simulink model "hamburger"  (R2021a)
settings: Solver=FixedStepAuto  StartTime=0.0  StopTime=150  FixedStep=0.1  RelTol=1e-3
settings Model: Creator=templ  LastModifiedBy=templ
settings DataIOCC: ReturnWorkspaceOutputs=off

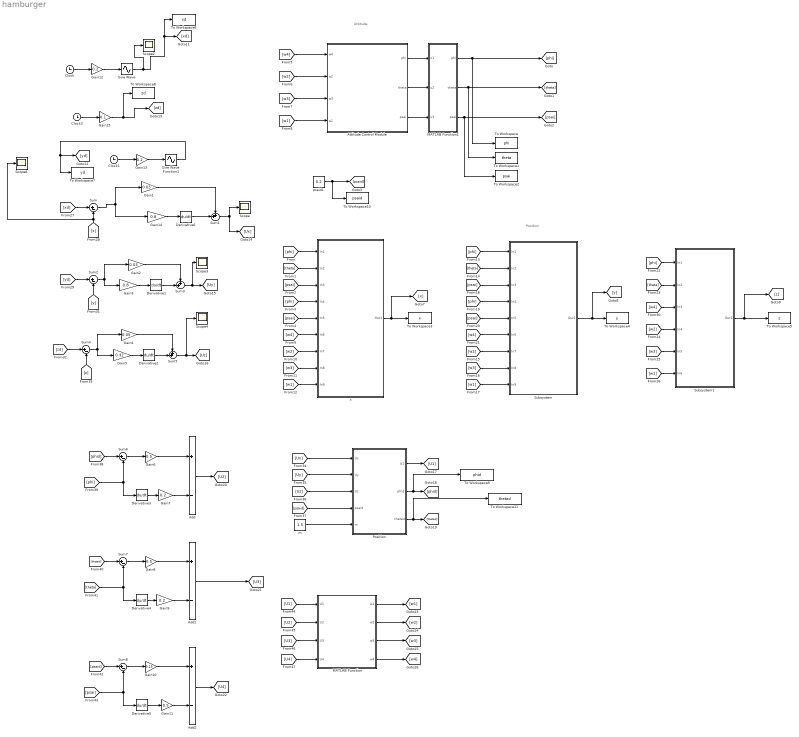
== system hamburger ==
  note: Attitude
  note: Position
  Add : Sum  Inputs=+-
  Add1 : Sum  Inputs=+-
  Add2 : Sum  Inputs=+-
  Attitude Control Module : Subsystem
  Clock : Clock
  Clock1 : Clock
  Clock3 : Clock
  Derivative{1..6} (6 alike) : Derivative
  Gain1 : Gain  Gain=0.03
  Gain10 : Gain  Gain=0.25
  Gain11 : Gain  Gain=0.5
  Gain{7,9,12..13} (4 alike) : Gain  Gain=0.2
  Gain14 : Gain  Gain=0.8
  Gain15 : Gain  Gain=0.1
  Gain2 : Gain  Gain=0.03
  Gain3 : Gain  Gain=0.8
  Gain4 : Gain  Gain=0.05
  Gain5 : Gain  Gain=0.32
  Gain6 : Gain  Gain=0.5
  Gain8 : Gain  Gain=0.5
  MATLAB Function : MATLAB Function  TreatAsAtomicUnit=on
  MATLAB Function1 : MATLAB Function  TreatAsAtomicUnit=on
  Position : MATLAB Function  TreatAsAtomicUnit=on
  Scope{,2..4,8} (5 alike) : Scope
  Sine Wave : Sin  TimeSource=Use external signal  Amplitude=2  SampleTime=0
  Sine Wave Function1 : Sin  TimeSource=Use external signal  Amplitude=2  Phase=pi/2  SampleTime=0
  Subsystem : Subsystem
  Subsystem1 : Subsystem
  Sum{,2,4,6..8} (6 alike) : Sum  Inputs=|+-
  Sum1 : Sum  Inputs=++|
  Sum3 : Sum  Inputs=++|
  Sum5 : Sum  Inputs=++|
  To Workspace : ToWorkspace  VariableName=phi  SampleTime=-1
  To Workspace1 : ToWorkspace  VariableName=theta  SampleTime=-1
  To Workspace10 : ToWorkspace  VariableName=psaid  SampleTime=-1
  To Workspace11 : ToWorkspace  VariableName=thetad  SampleTime=-1
  To Workspace2 : ToWorkspace  VariableName=psai  SampleTime=-1
  To Workspace3 : ToWorkspace  VariableName=x  SampleTime=-1
  To Workspace4 : ToWorkspace  VariableName=y  SampleTime=-1
  To Workspace5 : ToWorkspace  VariableName=z  SampleTime=-1
  To Workspace6 : ToWorkspace  VariableName=xd  SampleTime=-1
  To Workspace7 : ToWorkspace  VariableName=yd  SampleTime=-1
  To Workspace8 : ToWorkspace  VariableName=zd  SampleTime=-1
  To Workspace9 : ToWorkspace  VariableName=phid  SampleTime=-1
  m : Constant  Value=1.5
  psaid1 : Constant  Value=0.2
  x : Subsystem
  wires:
  [theta] -> Subsystem/2(In2)
  MATLAB Function/3(w3) -> [w3]
  Add2/1 -> [U4]
  [psaid] -> Sum8/1
  Gain8/1 -> Add1/1
  [U2] -> MATLAB Function/2(U2)
  [psai] -> Derivative5/1, Sum8/2
  [U1] -> MATLAB Function/1(U1)
  Sum2/1 -> Gain3/1, Gain2/1
  MATLAB Function/4(w4) -> [w4]
  [phid] -> Sum6/1
  Gain11/1 -> Add2/2
  [Uz] -> Position/3(Uz)
  [Ux] -> Position/1(Ux)
  [psaid] -> Position/4(psaid)
  x/1(Out1) -> [x], To Workspace3/1
  Position/1(U1) -> [U1]
  [w3] -> Subsystem/8(In8)
  m/1 -> Position/5(m)
  [w4] -> Subsystem/6(In6)
  [phi] -> Subsystem/4(In4)
  [w1] -> x/9(In9)
  Derivative3/1 -> Gain7/1
  Position/3(thetad) -> To Workspace11/1, [thetad]
  [theta] -> x/2(In2)
  [psai] -> Subsystem/5(In5)
  [w1] -> Subsystem1/6(In6)
  [w1] -> Attitude Control Module/4(w1)
  Attitude Control Module/3(psai) -> MATLAB Function1/3(u3)
  [w2] -> x/7(In7)
  [w3] -> Subsystem1/5(In5)
  [w4] -> Subsystem1/3(In3)
  Gain5/1 -> Derivative2/1
  [w2] -> Attitude Control Module/2(w2)
  Derivative2/1 -> Sum5/2
  MATLAB Function1/3(psai) -> To Workspace2/1, [psai]
  [w3] -> Attitude Control Module/3(w3)
  [psai] -> x/5(In5)
  [phi] -> Subsystem1/1(In1)
  [phi] -> x/4(In4)
  [psai] -> x/3(In3)
  [yd] -> Sum2/1
  Sum3/1 -> Scope3/1, [Uy]
  Derivative1/1 -> Sum3/2
  Gain2/1 -> Sum3/1
  [x] -> Scope8/1, Sum/2
  Clock/1 -> Gain12/1
  Clock3/1 -> Gain15/1
  Gain13/1 -> Sine Wave Function1/1
  [zd] -> Sum4/1
  Gain4/1 -> Sum5/1
  Gain15/1 -> [zd], To Workspace8/1
  [z] -> Sum4/2
  Gain3/1 -> Derivative1/1
  [U3] -> MATLAB Function/3(U3)
  [thetad] -> Sum7/1
  psaid1/1 -> To Workspace10/1, [psaid]
  [y] -> Sum2/2
  MATLAB Function1/1(phi) -> To Workspace/1, [phi]
  Sum7/1 -> Gain8/1
  [w2] -> Subsystem/7(In7)
  [w1] -> Subsystem/9(In9)
  Position/2(phid) -> To Workspace9/1, [phid]
  [U4] -> MATLAB Function/4(U4)
  Add/1 -> [U2]
  [phi] -> x/1(In1)
  Gain12/1 -> Sine Wave/1
  Gain7/1 -> Add/2
  Sum6/1 -> Gain6/1
  Attitude Control Module/2(theta) -> MATLAB Function1/2(u2)
  [w2] -> Subsystem1/4(In4)
  Subsystem/1(Out1) -> [y], To Workspace4/1
  MATLAB Function/2(w2) -> [w2]
  [xd] -> Sum/1
  Derivative5/1 -> Gain11/1
  MATLAB Function1/2(theta) -> To Workspace1/1, [theta]
  [Uy] -> Position/2(Uy)
  Sum4/1 -> Gain5/1, Gain4/1
  [phi] -> Derivative3/1, Sum6/2
  [theta] -> Subsystem1/2(In2)
  Add1/1 -> [U3]
  [w3] -> x/8(In8)
  Attitude Control Module/1(phi) -> MATLAB Function1/1(u1)
  [phi] -> Subsystem/1(In1)
  Clock1/1 -> Gain13/1
  Sum5/1 -> Scope4/1, [Uz]
  [psai] -> Subsystem/3(In3)
  [theta] -> Derivative4/1, Sum7/2
  Subsystem1/1(Out1) -> [z], To Workspace5/1
  Sine Wave/1 -> Scope2/1, To Workspace6/1, [xd]
  Derivative4/1 -> Gain9/1
  Gain9/1 -> Add1/2
  [w4] -> Attitude Control Module/1(w4)
  Gain10/1 -> Add2/1
  MATLAB Function/1(w1) -> [w1]
  Sum8/1 -> Gain10/1
  Gain6/1 -> Add/1
  Sum1/1 -> Scope/1, [Ux]
  [w4] -> x/6(In6)
  Sine Wave Function1/1 -> To Workspace7/1, [yd]
  Gain14/1 -> Derivative6/1
  Gain1/1 -> Sum1/1
  Derivative6/1 -> Sum1/2
  Sum/1 -> Gain14/1, Gain1/1

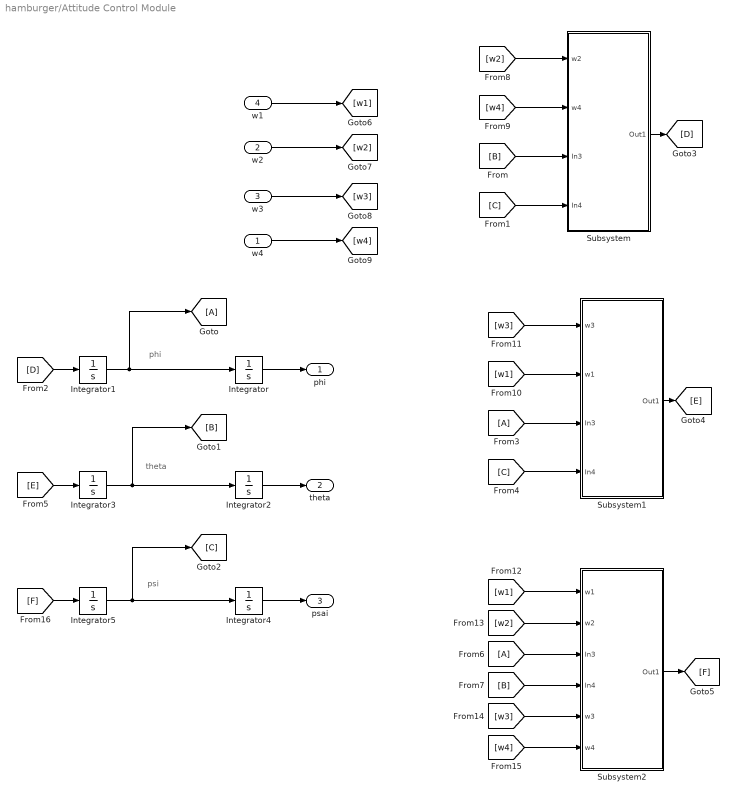
== system hamburger/Attitude Control Module ==
  note: phi
  note: theta
  note: psi
  w4 : Inport
  w2 : Inport  Port=2
  w3 : Inport  Port=3
  w1 : Inport  Port=4
  Integrator{,1..5} (6 alike) : Integrator
  Subsystem : Subsystem
  Subsystem1 : Subsystem
  Subsystem2 : Subsystem
  phi : Outport  VectorParamsAs1DForOutWhenUnconnected=off
  theta : Outport  Port=2  VectorParamsAs1DForOutWhenUnconnected=off
  psai : Outport  Port=3  VectorParamsAs1DForOutWhenUnconnected=off
  wires:
  [w2] -> Subsystem2/2(w2)
  [D] -> Integrator1/1
  [w1] -> Subsystem2/1(w1)
  Integrator1/1 -> [A], Integrator/1
  Subsystem2/1(Out1) -> [F]
  [C] -> Subsystem1/4(In4)
  [B] -> Subsystem2/4(In4)
  [A] -> Subsystem2/3(In3)
  Integrator3/1 -> [B], Integrator2/1
  [A] -> Subsystem1/3(In3)
  [C] -> Subsystem/4(In4)
  Subsystem1/1(Out1) -> [E]
  [w4] -> Subsystem2/6(w4)
  [F] -> Integrator5/1
  [w2] -> Subsystem/1(w2)
  [w4] -> Subsystem/2(w4)
  [w3] -> Subsystem2/5(w3)
  Integrator2/1 -> theta/1
  Subsystem/1(Out1) -> [D]
  Integrator5/1 -> [C], Integrator4/1
  Integrator/1 -> phi/1
  Integrator4/1 -> psai/1
  w4/1 -> [w4]
  w2/1 -> [w2]
  [B] -> Subsystem/3(In3)
  [E] -> Integrator3/1
  w1/1 -> [w1]
  w3/1 -> [w3]
  [w3] -> Subsystem1/1(w3)
  [w1] -> Subsystem1/2(w1)

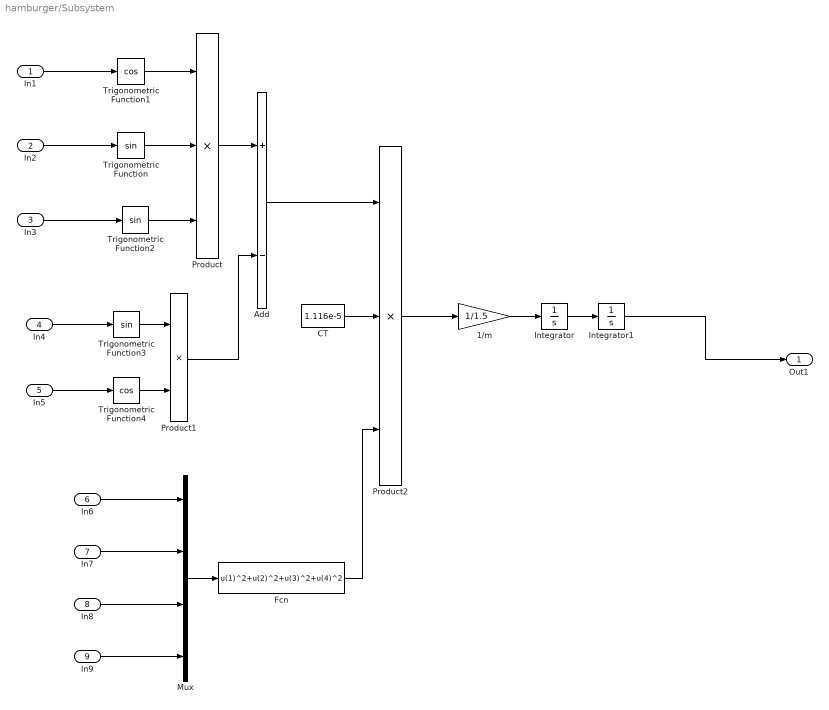
== system hamburger/Subsystem ==
  In1 : Inport
  In2 : Inport  Port=2
  In3 : Inport  Port=3
  In4 : Inport  Port=4
  In5 : Inport  Port=5
  In6 : Inport  Port=6
  In7 : Inport  Port=7
  In8 : Inport  Port=8
  In9 : Inport  Port=9
  1/m : Gain  Gain=1/1.5
  Add : Sum  Inputs=+-
  CT : Constant  Value=1.116e-5
  Fcn : Fcn  Expr=u(1)^2+u(2)^2+u(3)^2+u(4)^2
  Integrator : Integrator
  Integrator1 : Integrator
  Mux : Mux
  Product : Product  Inputs=3
  Product1 : Product
  Product2 : Product  Inputs=3
  Trigonometric Function : Trigonometry
  Trigonometric Function1 : Trigonometry  Operator=cos
  Trigonometric Function2 : Trigonometry
  Trigonometric Function3 : Trigonometry
  Trigonometric Function4 : Trigonometry  Operator=cos
  Out1 : Outport  VectorParamsAs1DForOutWhenUnconnected=off
  wires:
  Mux/1 -> Fcn/1
  Product2/1 -> 1/m/1
  Fcn/1 -> Product2/3
  CT/1 -> Product2/2
  Trigonometric Function2/1 -> Product/3
  Trigonometric Function/1 -> Product/2
  Trigonometric Function3/1 -> Product1/1
  Product1/1 -> Add/2
  Product/1 -> Add/1
  Add/1 -> Product2/1
  In4/1 -> Trigonometric Function3/1
  Trigonometric Function1/1 -> Product/1
  Integrator/1 -> Integrator1/1
  In8/1 -> Mux/3
  Trigonometric Function4/1 -> Product1/2
  1/m/1 -> Integrator/1
  Integrator1/1 -> Out1/1
  In9/1 -> Mux/4
  In1/1 -> Trigonometric Function1/1
  In6/1 -> Mux/1
  In5/1 -> Trigonometric Function4/1
  In7/1 -> Mux/2
  In3/1 -> Trigonometric Function2/1
  In2/1 -> Trigonometric Function/1

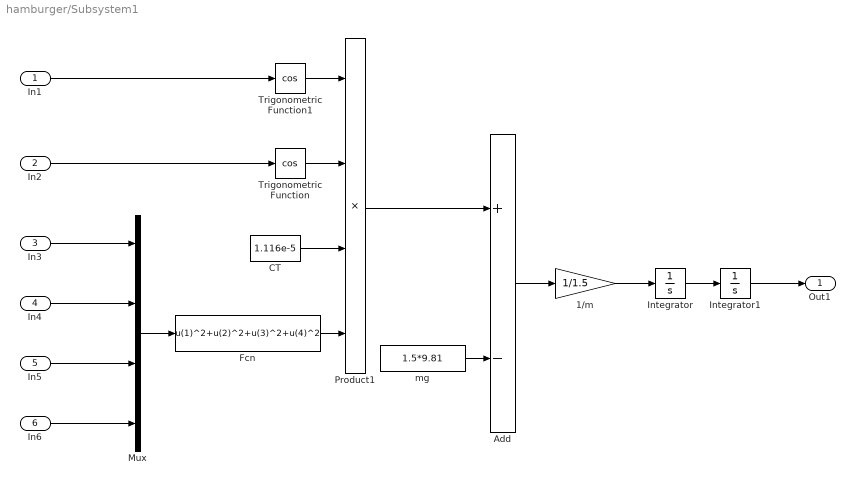
== system hamburger/Subsystem1 ==
  In1 : Inport
  In2 : Inport  Port=2
  In3 : Inport  Port=3
  In4 : Inport  Port=4
  In5 : Inport  Port=5
  In6 : Inport  Port=6
  1/m : Gain  Gain=1/1.5
  Add : Sum  Inputs=+-
  CT : Constant  Value=1.116e-5
  Fcn : Fcn  Expr=u(1)^2+u(2)^2+u(3)^2+u(4)^2
  Integrator : Integrator
  Integrator1 : Integrator
  Mux : Mux
  Product1 : Product  Inputs=4
  Trigonometric Function : Trigonometry  Operator=cos
  Trigonometric Function1 : Trigonometry  Operator=cos
  mg : Constant  Value=1.5*9.81
  Out1 : Outport  VectorParamsAs1DForOutWhenUnconnected=off
  wires:
  Trigonometric Function1/1 -> Product1/1
  Integrator/1 -> Integrator1/1
  Fcn/1 -> Product1/4
  mg/1 -> Add/2
  CT/1 -> Product1/3
  Add/1 -> 1/m/1
  Mux/1 -> Fcn/1
  In2/1 -> Trigonometric Function/1
  1/m/1 -> Integrator/1
  Trigonometric Function/1 -> Product1/2
  Product1/1 -> Add/1
  In4/1 -> Mux/2
  Integrator1/1 -> Out1/1
  In5/1 -> Mux/3
  In3/1 -> Mux/1
  In6/1 -> Mux/4
  In1/1 -> Trigonometric Function1/1

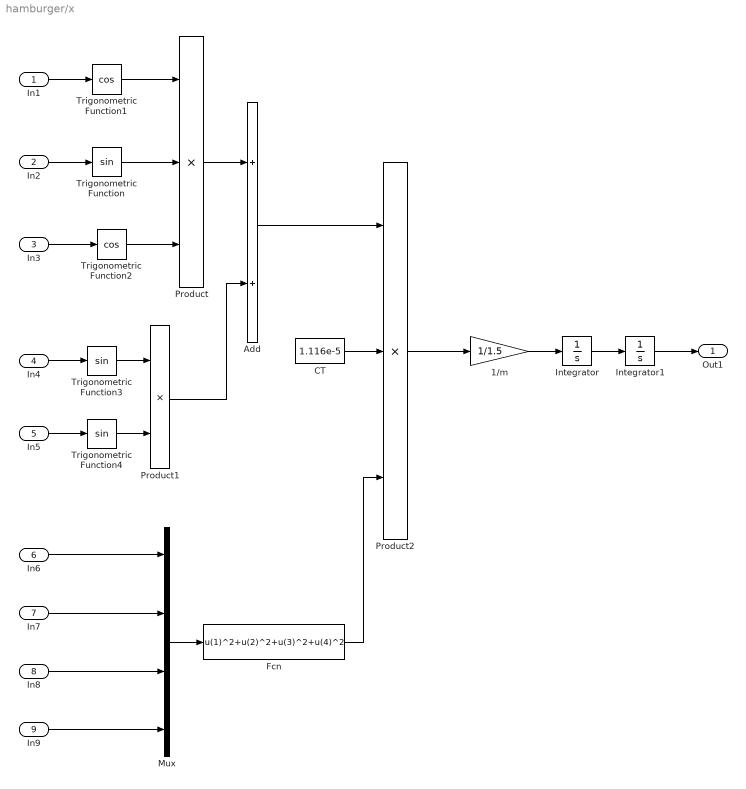
== system hamburger/x ==
  In1 : Inport
  In2 : Inport  Port=2
  In3 : Inport  Port=3
  In4 : Inport  Port=4
  In5 : Inport  Port=5
  In6 : Inport  Port=6
  In7 : Inport  Port=7
  In8 : Inport  Port=8
  In9 : Inport  Port=9
  1/m : Gain  Gain=1/1.5
  Add : Sum
  CT : Constant  Value=1.116e-5
  Fcn : Fcn  Expr=u(1)^2+u(2)^2+u(3)^2+u(4)^2
  Integrator : Integrator
  Integrator1 : Integrator
  Mux : Mux
  Product : Product  Inputs=3
  Product1 : Product
  Product2 : Product  Inputs=3
  Trigonometric Function : Trigonometry
  Trigonometric Function1 : Trigonometry  Operator=cos
  Trigonometric Function2 : Trigonometry  Operator=cos
  Trigonometric Function3 : Trigonometry
  Trigonometric Function4 : Trigonometry
  Out1 : Outport  VectorParamsAs1DForOutWhenUnconnected=off
  wires:
  In8/1 -> Mux/3
  Integrator1/1 -> Out1/1
  1/m/1 -> Integrator/1
  Trigonometric Function4/1 -> Product1/2
  Integrator/1 -> Integrator1/1
  In7/1 -> Mux/2
  Add/1 -> Product2/1
  Product1/1 -> Add/2
  Product/1 -> Add/1
  In4/1 -> Trigonometric Function3/1
  Fcn/1 -> Product2/3
  Trigonometric Function1/1 -> Product/1
  In2/1 -> Trigonometric Function/1
  Trigonometric Function/1 -> Product/2
  Trigonometric Function2/1 -> Product/3
  Trigonometric Function3/1 -> Product1/1
  CT/1 -> Product2/2
  In1/1 -> Trigonometric Function1/1
  Product2/1 -> 1/m/1
  In3/1 -> Trigonometric Function2/1
  Mux/1 -> Fcn/1
  In6/1 -> Mux/1
  In5/1 -> Trigonometric Function4/1
  In9/1 -> Mux/4

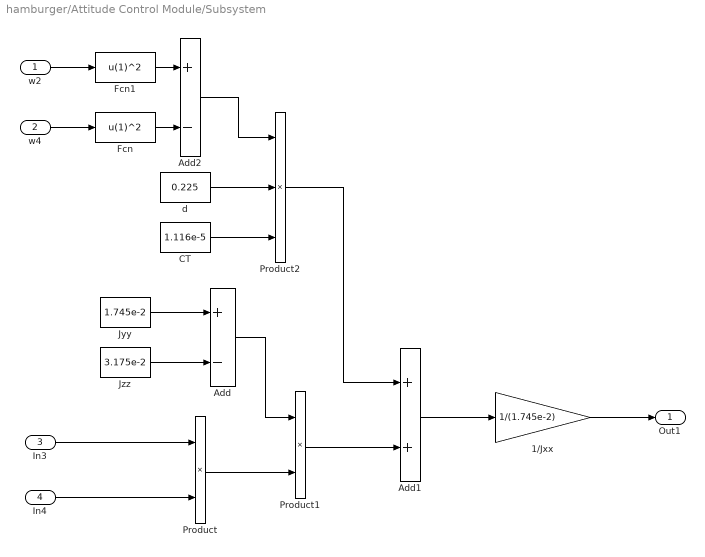
== system hamburger/Attitude Control Module/Subsystem ==
  w2 : Inport
  w4 : Inport  Port=2
  In3 : Inport  Port=3
  In4 : Inport  Port=4
  1/Jxx : Gain  Gain=1/(1.745e-2)
  Add : Sum  Inputs=+-
  Add1 : Sum
  Add2 : Sum  Inputs=+-
  CT : Constant  Value=1.116e-5
  Fcn : Fcn  Expr=u(1)^2
  Fcn1 : Fcn  Expr=u(1)^2
  Jyy : Constant  Value=1.745e-2
  "Jzz " : Constant  Value=3.175e-2
  Product : Product
  Product1 : Product
  Product2 : Product  Inputs=3
  d : Constant  Value=0.225
  Out1 : Outport  VectorParamsAs1DForOutWhenUnconnected=off
  wires:
  Product2/1 -> Add1/1
  Fcn/1 -> Add2/2
  CT/1 -> Product2/3
  "Jzz "/1 -> Add/2
  Add1/1 -> 1/Jxx/1
  Fcn1/1 -> Add2/1
  Add2/1 -> Product2/1
  Product1/1 -> Add1/2
  Product/1 -> Product1/2
  d/1 -> Product2/2
  In4/1 -> Product/2
  Jyy/1 -> Add/1
  w4/1 -> Fcn/1
  Add/1 -> Product1/1
  1/Jxx/1 -> Out1/1
  w2/1 -> Fcn1/1
  In3/1 -> Product/1

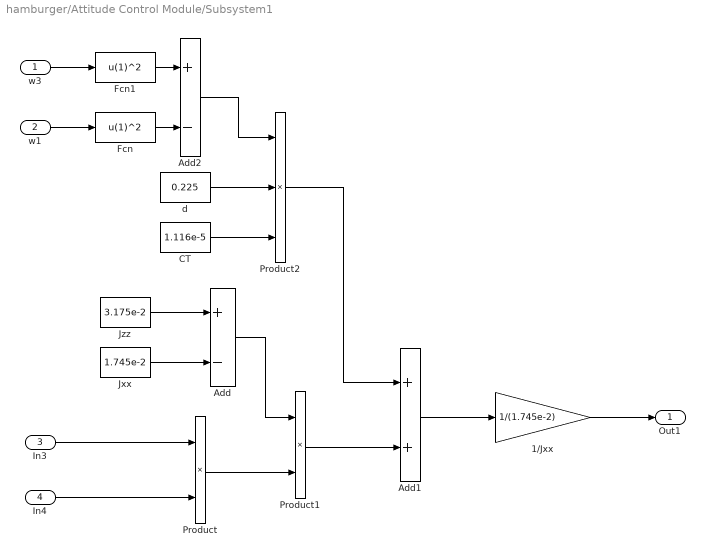
== system hamburger/Attitude Control Module/Subsystem1 ==
  w3 : Inport
  w1 : Inport  Port=2
  In3 : Inport  Port=3
  In4 : Inport  Port=4
  1/Jxx : Gain  Gain=1/(1.745e-2)
  Add : Sum  Inputs=+-
  Add1 : Sum
  Add2 : Sum  Inputs=+-
  CT : Constant  Value=1.116e-5
  Fcn : Fcn  Expr=u(1)^2
  Fcn1 : Fcn  Expr=u(1)^2
  Jxx : Constant  Value=1.745e-2
  Jzz : Constant  Value=3.175e-2
  Product : Product
  Product1 : Product
  Product2 : Product  Inputs=3
  d : Constant  Value=0.225
  Out1 : Outport  VectorParamsAs1DForOutWhenUnconnected=off
  wires:
  Product2/1 -> Add1/1
  Fcn/1 -> Add2/2
  CT/1 -> Product2/3
  Jxx/1 -> Add/2
  Add1/1 -> 1/Jxx/1
  Fcn1/1 -> Add2/1
  Add2/1 -> Product2/1
  Product1/1 -> Add1/2
  Product/1 -> Product1/2
  d/1 -> Product2/2
  In4/1 -> Product/2
  Jzz/1 -> Add/1
  w1/1 -> Fcn/1
  Add/1 -> Product1/1
  1/Jxx/1 -> Out1/1
  w3/1 -> Fcn1/1
  In3/1 -> Product/1

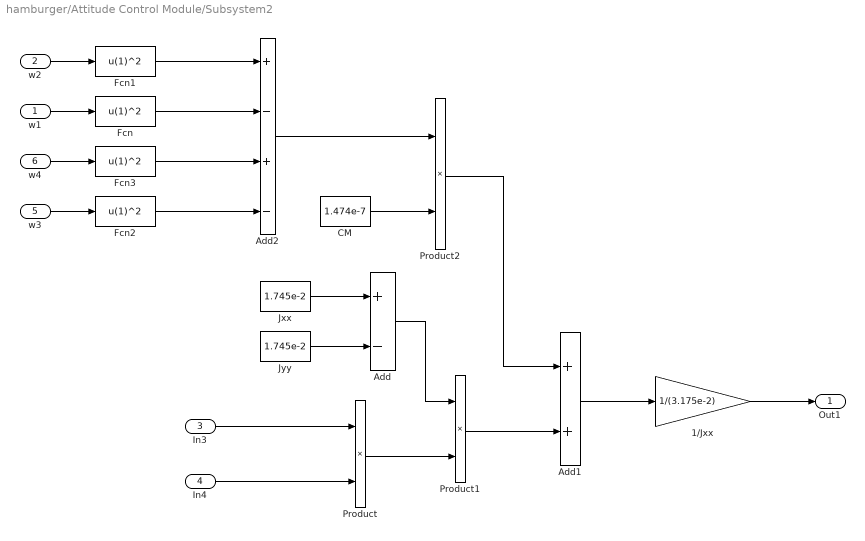
== system hamburger/Attitude Control Module/Subsystem2 ==
  w1 : Inport
  w2 : Inport  Port=2
  In3 : Inport  Port=3
  In4 : Inport  Port=4
  w3 : Inport  Port=5
  w4 : Inport  Port=6
  1/Jxx : Gain  Gain=1/(3.175e-2)
  Add : Sum  Inputs=+-
  Add1 : Sum
  Add2 : Sum  Inputs=+-+-
  CM : Constant  Value=1.474e-7
  Fcn{,1..3} (4 alike) : Fcn  Expr=u(1)^2
  Jxx : Constant  Value=1.745e-2
  Jyy : Constant  Value=1.745e-2
  Product : Product
  Product1 : Product
  Product2 : Product
  Out1 : Outport  VectorParamsAs1DForOutWhenUnconnected=off
  wires:
  Product2/1 -> Add1/1
  CM/1 -> Product2/2
  Jyy/1 -> Add/2
  Add1/1 -> 1/Jxx/1
  Add2/1 -> Product2/1
  Product1/1 -> Add1/2
  Product/1 -> Product1/2
  In4/1 -> Product/2
  Jxx/1 -> Add/1
  Add/1 -> Product1/1
  1/Jxx/1 -> Out1/1
  In3/1 -> Product/1
  Fcn1/1 -> Add2/1
  Fcn/1 -> Add2/2
  Fcn3/1 -> Add2/3
  Fcn2/1 -> Add2/4
  w2/1 -> Fcn1/1
  w4/1 -> Fcn3/1
  w1/1 -> Fcn/1
  w3/1 -> Fcn2/1

== matlab function hamburger/MATLAB Function ==
  data: U1 input; w1 output; U2 input; U3 input; U4 input; w2 output; w3 output; w4 output
function [w1,w2,w3,w4] = fcn(U1,U2,U3,U4)
    CT = 1.116e-5; dCT = 0.225*CT;
    matrixA = [CT,CT,CT,CT;0,CT,0,-CT;-CT,0,CT,0;-dCT,dCT,-dCT,dCT];
    w_2 = inv(matrixA)*[U1,U2,U3,U4]';
    w1 = sqrt(abs(w_2(1))); w2 = sqrt(abs(w_2(2)));
    w3 = sqrt(abs(w_2(3))); w4 = sqrt(abs(w_2(4)));
end

== matlab function hamburger/Position ==
  data: Ux input; U1 output; Uy input; Uz input; psaid input; m input; phid output; thetad output
function [U1,phid,thetad] = fcn(Ux,Uy,Uz,psaid,m)
    U1 = m*sqrt(Ux^2+Uy^2+(Uz+9.81)^2);
    phid = asin((Ux*sin(psaid)-Uy*cos(psaid))*m/U1);
    thetad = asin((Ux*m-U1*sin(psaid)*sin(phid))/(U1*cos(psaid)*cos(phid)));
end

== matlab function hamburger/MATLAB Function1 ==
  data: u1 input; phi output; u2 input; u3 input; theta output; psai output
function [phi,theta,psai] = fcn(u1,u2,u3)
    phi = rem(u1,2*pi);
    theta = rem(u2,2*pi);
    psai = rem(u3,2*pi);
end
